simulink model "buck_converter_DE_Parallel_Plecs"  (R2023b)
settings: Solver=VariableStepAuto  StartTime=0.0  StopTime=Tend  RelTol=1e-3
values from neighbouring files (symbols this model uses):
  Ki = Ki_best    [main.m]    (also in main_DE_Parallel.m)
  Kp = Kp_best    [main.m]    (also in main_DE_Parallel.m)
  Tsamp = 1/Fsamp    (= 1e-06)    [main.m]    (also in main_DE_Parallel.m)
  Ttrig = Tend/2    (= 0.05)    [main.m]    (also in main_DE_Parallel.m)
  Vref1 = 40    [main.m]    (also in main_DE_Parallel.m)
  Vref2 = 60    [main.m]    (also in main_DE_Parallel.m)
undefined symbols (not defined in the file or in its folder): plecs
libraries: simulink_extras x1, sps_lib x1
settings Model: Creator=baik3-ad  LastModifiedBy=baik3-ad

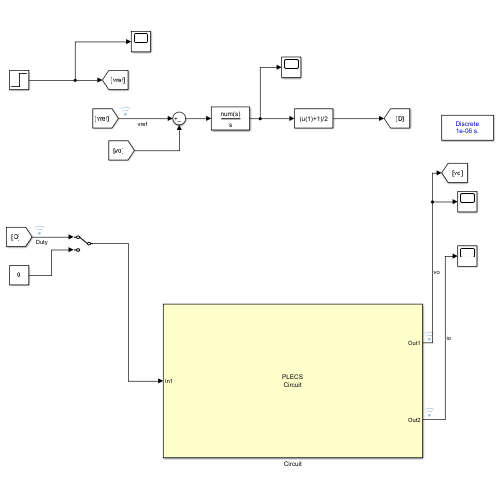
[thumbnail: Simulink's stored preview of the top-level diagram]
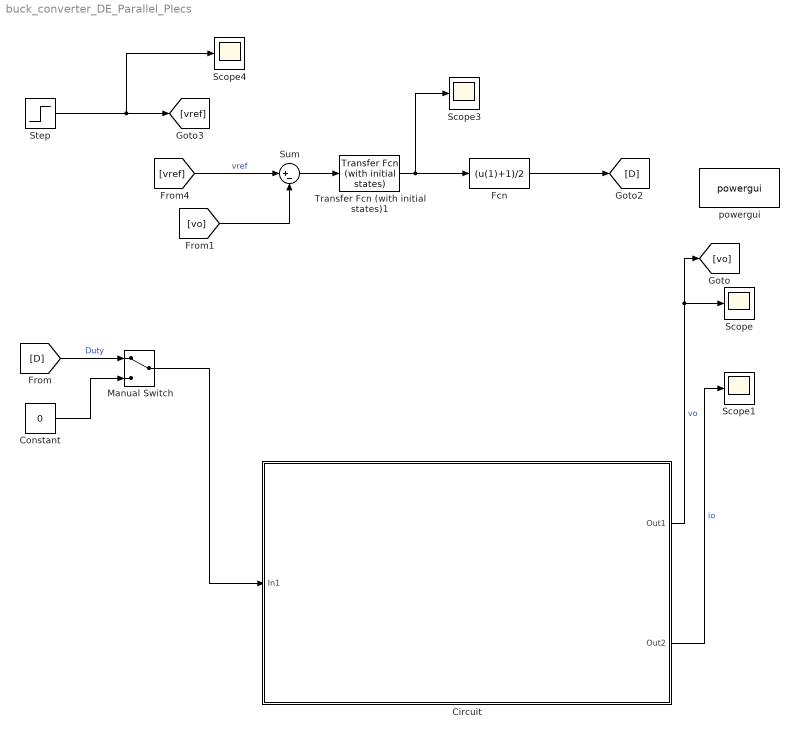
== system buck_converter_DE_Parallel_Plecs ==
  Circuit : Subsystem  LoadFcn=plecs('sl', 200);  InitFcn=plecs('sl', 214);  StartFcn=plecs('sl', 208);  StopFcn=plecs('sl', 209);  mask(PlecsCircuit){PLECSData=<binary blob, 3324 chars, not shown>}
      mask prompts: PLECSData "PLECS Data (Do not delete or modify!)"
      mask init:
      | % PLACE CUSTOM INITIALIZATIONS ABOVE
      | % DO NOT REMOVE
      | plecs('sl', 215);
      | % DO NOT REMOVE
      settings: CopyFcn=plecs('sl', 203);  DeleteFcn=plecs('sl', 205);  UndoDeleteFcn=plecs('sl', 206);  PreSaveFcn=plecs('sl', 211);  PostSaveFcn=plecs('sl', 201);  NameChangeFcn=plecs('sl', 210);  DestroyFcn=plecs('sl', 207);  PreCopyFcn=plecs('sl', 216);  OpenFcn=plecs('sl', 202);  ErrorFcn=plerrorfcn
      mask Help: eval('plecs(''help'', ''qthelp:///creatingacircuit.html'')')
      mask Display: disp('PLECS\nCircuit')
  Constant : Constant  Value=0
  Fcn : Fcn  Expr=(u(1)+1)/2
  Manual Switch : ManualSwitch
  Scope{,1,3..4} (4 alike) : Scope
  Step : Step  Time=Ttrig  Before=Vref1  After=Vref2  SampleTime=Tsamp
  Sum : Sum  Inputs=|+-
  Transfer Fcn (with initial states)1 : simulink_extras/Additional Linear/Transfer Fcn (with initial states)  N=[Kp Ki]  D="[1  0]"  X0=0
  powergui : sps_lib/powergui  Priority=1  SimulationMode=Discrete  SampleTime=Tsamp  frequency=60  Iterations=50  frequencyindice=0  Pbase=100e6  ErrMax=1e-4  UnitsV=kV  UnitsW=MW  buscounter=0  FunctionMessages=off  echomessages=off  EnableUseOfTLC=off  CurrentSourceSwitches=off  DisableSnubberDevices=off  DisableRonSwitches=off  DisableVfSwitches=off  DisplayEquations=off  AutomaticDiscreteSolvers=off  SolverType=Tustin/Backward Euler (TBE)  Interpol=off  ExternalGateDelay=off  methode=off  Ts=100  x0status=blocks  SPID=on  SwTol=0  HookPort=off  NonlinearTolerance=1e-4  nMaxIteration=100  ContinueOnMaxIteration=off  RestoreLinks=warning  ResistiveCurrentMeasurement=off  Frange=[0:2:500]  Ylog=off  Xlog=on  ShowGrid=off  save=off  variable=ZData  structure=0  ZoomFFT=off  StartTime=0.0  cycles=1  DisplayStyle=1  fundamental=60  FreqAxis=off  MaxFrequency=1000  frequencyindicesteady=1  RmsSteady=1  display=off
  wires:
  [vref] -> Sum/1  "vref"
  Sum/1 -> Transfer Fcn (with initial states)1/1
  Step/1 -> Scope4/1, [vref]
  Transfer Fcn (with initial states)1/1 -> Fcn/1, Scope3/1
  [vo] -> Sum/2
  Circuit/1(Out1) -> Scope/1, [vo]  "vo"
  Circuit/2(Out2) -> Scope1/1  "io"
  [D] -> Manual Switch/1  "Duty"
  Constant/1 -> Manual Switch/2
  Manual Switch/1 -> Circuit/1(In1)
  Fcn/1 -> [D]

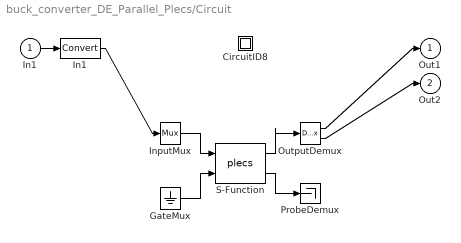
== system buck_converter_DE_Parallel_Plecs/Circuit ==
  In1 : Inport  PortDimensions=1
  " CircuitID8 " : Subsystem
  " GateMux " : Ground
  " In1 " : DataTypeConversion
  " InputMux " : Mux  Inputs=[ 1 ]
  " OutputDemux " : Demux  Outputs=[ 1 1 ]
  " ProbeDemux " : Terminator
  " S-Function " : S-Function  FunctionName=plecs  SFunctionDeploymentMode=off  EnableBusSupport=off
  Out1 : Outport  PortDimensions=1
  Out2 : Outport  Port=2  PortDimensions=1
  wires:
  " S-Function "/1 -> " OutputDemux "/1
  " InputMux "/1 -> " S-Function "/1
  " GateMux "/1 -> " S-Function "/2
  " S-Function "/2 -> " ProbeDemux "/1
  In1/1 -> " In1 "/1
  " In1 "/1 -> " InputMux "/1
  " OutputDemux "/1 -> Out1/1
  " OutputDemux "/2 -> Out2/1

== system buck_converter_DE_Parallel_Plecs/Circuit/ CircuitID8  ==
